simulink model "q_loop_uncontrolled"  (R2019a)
settings: Solver=ode45  StartTime=0.0  StopTime=10.0  MaxStep=0.01  RelTol=1e-3
values from neighbouring files (symbols this model uses):
  A = SS_long.A    [PlacePoles.m]
  B = SS_long.B(:, 2)    [PlacePoles.m]
  C_c = eye(2)    [PlacePoles.m]
  D_c = D    [PlacePoles.m]
  Ka = F(1)    [PlacePoles.m]
  Kq = F(2)    [PlacePoles.m]
libraries: cstblocks x2, simulink_extras x2
settings Model: Creator=tblaha  LastModifiedBy=tblaha
settings SolverCC: SolverOrder=5

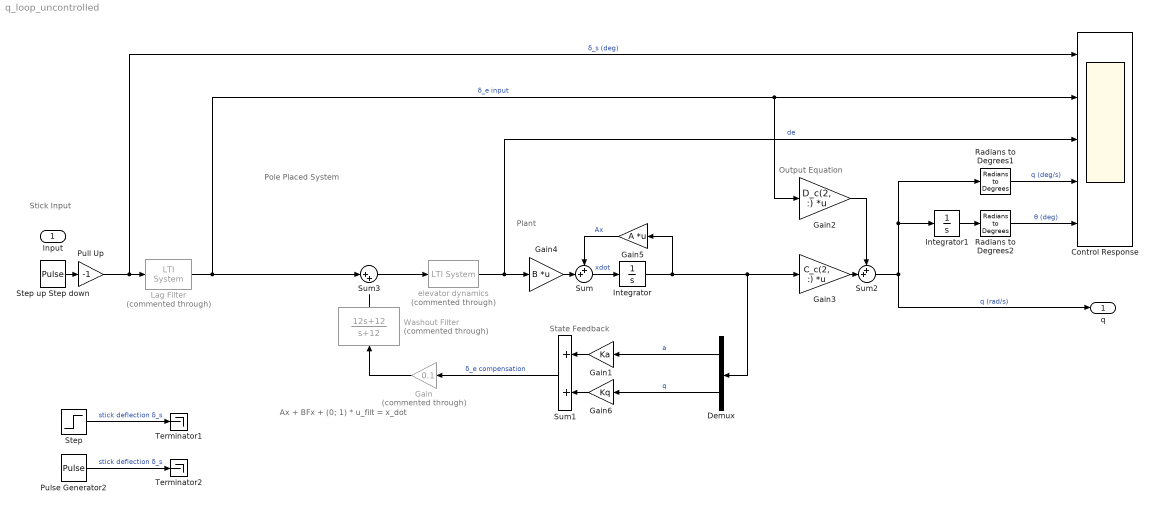
== system q_loop_uncontrolled ==
  note: Plant
  note: State Feedback
  note: Output Equation
  note: Stick Input
  note: Pole Placed System
  note: Ax + BFx + (0; 1) * u_filt = x_dot
  Input : Inport
  Control Response : Scope  NumInputPorts=5
  Demux : Demux  Outputs=2
  Gain : Gain  Commented=through  Gain=0.1
  Gain1 : Gain  Gain=Ka
  Gain2 : Gain  Gain=D_c(2, :)  Multiplication=Matrix(K*u)
  Gain3 : Gain  Gain=C_c(2, :)  Multiplication=Matrix(K*u)
  Gain4 : Gain  Gain=B  Multiplication=Matrix(K*u)
  Gain5 : Gain  Gain=A  Multiplication=Matrix(K*u)
  Gain6 : Gain  Gain=Kq
  Integrator : Integrator  InitialCondition=[0 0]
  Integrator1 : Integrator
  Lag Filter : cstblocks/LTI System  Commented=through  sys=LL_filt  IC=[]
  Pull Up : Gain  Gain=-1
  Pulse Generator2 : DiscretePulseGenerator  PulseType=Time based  Period=10  PulseWidth=60  PhaseDelay=1
  Radians to Degrees1 : simulink_extras/Transformations/Radians to Degrees
  Radians to Degrees2 : simulink_extras/Transformations/Radians to Degrees
  Step : Step  After=10  SampleTime=0
  Step up Step down : DiscretePulseGenerator  PulseType=Time based  Period=10  PulseWidth=60  PhaseDelay=1
  Sum : Sum  Inputs=++|
  Sum1 : Sum
  Sum2 : Sum  Inputs=++|
  Sum3 : Sum  Inputs=|++
  Terminator1 : Terminator
  Terminator2 : Terminator
  Washout Filter : TransferFcn  Commented=through  Numerator=[12 12]  Denominator=[1 12]
  elevator dynamics : cstblocks/LTI System  Commented=through  sys=H_servo  IC=[]
  q : Outport
  wires:
  Gain2/1 -> Sum2/1
  Sum2/1 -> Radians to Degrees1/1, Integrator1/1, q/1  "q (rad/s)"
  Step up Step down/1 -> Pull Up/1
  Demux/1 -> Gain1/1  "a"
  Demux/2 -> Gain6/1  "q"
  Gain1/1 -> Sum1/1
  Gain6/1 -> Sum1/2
  Gain3/1 -> Sum2/2
  Lag Filter/1 -> Control Response/2, Gain2/1, Sum3/1  "δ_e input"
  Radians to Degrees1/1 -> Control Response/4  "q (deg/s)"
  Integrator1/1 -> Radians to Degrees2/1
  Radians to Degrees2/1 -> Control Response/5  "θ (deg)"
  Step/1 -> Terminator1/1  "stick deflection δ_s"
  Pulse Generator2/1 -> Terminator2/1  "stick deflection δ_s"
  Integrator/1 -> Gain3/1, Demux/1, Gain5/1
  Sum1/1 -> Gain/1  "δ_e compensation"
  elevator dynamics/1 -> Control Response/3, Gain4/1  "de"
  Sum3/1 -> elevator dynamics/1
  Washout Filter/1 -> ?
  Gain/1 -> Washout Filter/1
  Gain4/1 -> Sum/2
  Gain5/1 -> Sum/1  "Ax"
  Sum/1 -> Integrator/1  "xdot"
  Pull Up/1 -> Lag Filter/1, Control Response/1  "δ_s (deg)"
